simulink model "Final_PV1"  (R2015a)
settings: Solver=ode45  StartTime=0.0  StopTime=.08  MinStep=.00001  RelTol=1e-6
undefined symbols (not defined in the file): sigbuilder_block
libraries: powerlib x8, simulink x2
settings Model: Creator=TCM  LastModifiedBy=pc
settings SolverCC: ZeroCrossControl=EnableAll
settings DebuggingCC: UnderspecifiedInitializationDetection=Classic  MergeDetectMultiDrivingBlocksExec=none  SolverPrmCheckMsg=warning  StateNameClashWarn=warning

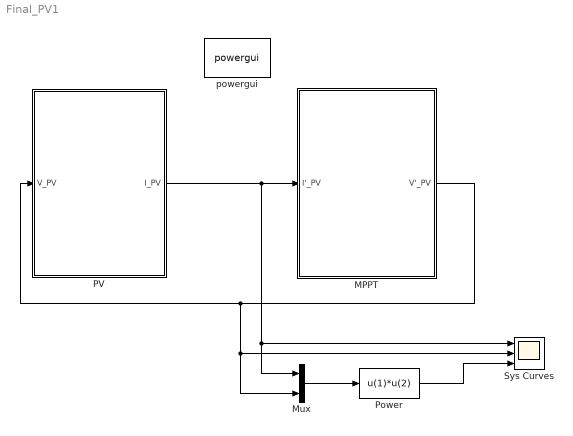
== system Final_PV1 ==
  MPPT : Subsystem
  Mux : Mux  Inputs=2
  PV : Subsystem
  "Power " : Fcn  Expr=u(1)*u(2)
  Sys Curves : Scope  NumInputPorts=3
      settings: YMin=0~0~6.15  YMax=400~80~6.4  SaveName=ScopeData2
  powergui : powerlib/powergui  Priority=1  SimulationMode=Discrete  SolverType=Tustin  SampleTime=50e-6  frequency=60  SPID=on  DisableSnubberDevices=off  DisableRonSwitches=off  DisableVfSwitches=off  SwTol=0  DisplayEquations=off  Interpol=off  methode=off  Ts=100  FunctionMessages=off  echomessages=off  HookPort=off  EnableUseOfTLC=off  x0status=blocks  frequencyindice=0  Pbase=100e6  ErrMax=1e-4  Iterations=50  UnitsV=kV  UnitsW=MW  buscounter=0  RestoreLinks=warning  ResistiveCurrentMeasurement=off  Frange=[0:2:500]  Ylog=off  Xlog=on  ShowGrid=off  save=off  variable=ZData  structure=0  ZoomFFT=off  StartTime=0.0  cycles=1  DisplayStyle=1  fundamental=60  FreqAxis=off  MaxFrequency=1000  frequencyindicesteady=1  RmsSteady=1  display=off
  wires:
  PV/1(I_PV) -> MPPT/1(I'_PV), Sys Curves/1, Mux/1
  Mux/1 -> "Power "/1
  "Power "/1 -> Sys Curves/3
  MPPT/1("V'_PV ") -> Mux/2, Sys Curves/2, PV/1(V_PV)

== system Final_PV1/MPPT ==
  I'_PV : Inport
  "MPPT " : Subsystem
  "V'_PV " : Outport
  wires:
  "MPPT "/1(V_mpp) -> "V'_PV "/1, "MPPT "/2(V_PV)
  I'_PV/1 -> "MPPT "/1(I_PV)

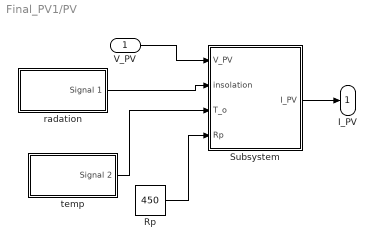
== system Final_PV1/PV ==
  V_PV : Inport
  Rp : Constant  Value=450
  Subsystem : Subsystem
  radation : Subsystem  Tag=STV Subsys  LoadFcn=sigbuilder_block('load');  StartFcn=sigbuilder_block('start');  StopFcn=sigbuilder_block('stop');  ClipboardFcn=sigbuilder_block('clipboard');  mask(Sigbuilder block){}
      mask help: Simulink:masks:SigbuilderBlock_MD
      mask init:
      | if ~strcmp(get_param(bdroot(gcbh),'SimulationStatus'),'stopped') tuvar = sigbuilder_block('maskInit'); end
      settings: CopyFcn=sigbuilder_block('copy');  DeleteFcn=sigbuilder_block('delete');  ModelCloseFcn=sigbuilder_block('modelClose');  PreSaveFcn=sigbuilder_block('preSave');  PauseFcn=sigbuilder_block('pause');  ContinueFcn=sigbuilder_block('continue');  NameChangeFcn=sigbuilder_block('namechange');  OpenFcn=sigbuilder_block('open',[267 58.5 550.5 394.5 ]);  CloseFcn=sigbuilder_block('close');
      mask Display: plot(0, 0, 100, 100,[2, 2, 32, 32, 2], [68, 8, 8, 68, 68],[32, 2], [38, 38], [32, 19, 2],[53, 60, 44], [32, 17, 17, 2],[16, 16, 31, 31]);txt = getActiveGroup(gcbh);text(2, 100, txt,'verticalAlignment', 'top');
  temp : Subsystem  Tag=STV Subsys  LoadFcn=sigbuilder_block('load');  StartFcn=sigbuilder_block('start');  StopFcn=sigbuilder_block('stop');  ClipboardFcn=sigbuilder_block('clipboard');  mask(Sigbuilder block){}
      mask help: Simulink:masks:SigbuilderBlock_MD
      mask init:
      | if ~strcmp(get_param(bdroot(gcbh),'SimulationStatus'),'stopped') tuvar = sigbuilder_block('maskInit'); end
      settings: CopyFcn=sigbuilder_block('copy');  DeleteFcn=sigbuilder_block('delete');  ModelCloseFcn=sigbuilder_block('modelClose');  PreSaveFcn=sigbuilder_block('preSave');  PauseFcn=sigbuilder_block('pause');  ContinueFcn=sigbuilder_block('continue');  NameChangeFcn=sigbuilder_block('namechange');  OpenFcn=sigbuilder_block('open',[437.25 118.5 550.5 394.5 ]);  CloseFcn=sigbuilder_block('close');
      mask Display: plot(0, 0, 100, 100,[2, 2, 32, 32, 2], [68, 8, 8, 68, 68],[32, 2], [38, 38], [32, 19, 2],[53, 60, 44], [32, 17, 17, 2],[16, 16, 31, 31]);txt = getActiveGroup(gcbh);text(2, 100, txt,'verticalAlignment', 'top');
  I_PV : Outport
  wires:
  Subsystem/1(I_PV) -> I_PV/1
  temp/1(Signal 2) -> Subsystem/3(T_o)
  radation/1(Signal 1) -> Subsystem/2(insolation)
  Rp/1 -> Subsystem/4(Rp)
  V_PV/1 -> Subsystem/1(V_PV)

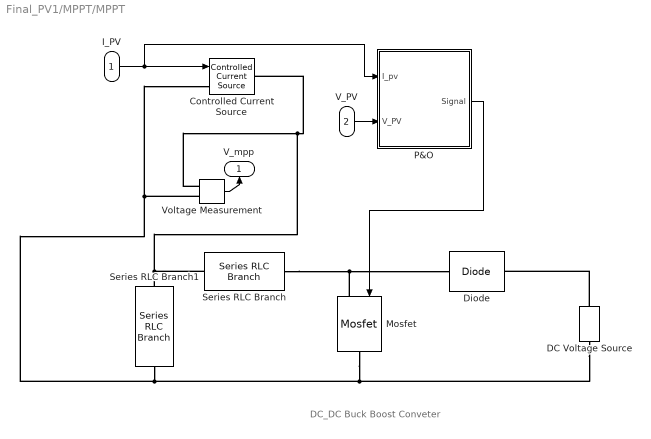
== system Final_PV1/MPPT/MPPT  ==
  note: DC_DC Buck Boost Conveter
  I_PV : Inport
  V_PV : Inport  Port=2
  Controlled Current Source : powerlib/Electrical Sources/Controlled Current Source  Initialize=on  Source_Type=AC  Amplitude=0  Phase=0  Frequency=0  Measurements=None
  DC Voltage Source : powerlib/Electrical Sources/DC Voltage Source  Amplitude=55  Measurements=None
  Diode : powerlib/Power Electronics/Diode  Ron=0.001  Lon=0  Vf=0.8  IC=0  UseSnubber=off  Rs=500  Cs=250e-9  Measurements=off
  Mosfet : powerlib/Power Electronics/Mosfet  Ron=0.1  Lon=0  Rd=0.01  Vfd=0  IC=0  Rs=1e5  Cs=inf  Measurements=off
  "P&O " : Subsystem
  Series RLC Branch : powerlib/Elements/Series RLC Branch  LConnTagsString=__new0  RConnTagsString=__new0  BranchType=RL  Resistance=.45  Inductance=1e-3  SetiL0=off  InitialCurrent=0  Capacitance=1e-6  Setx0=off  InitialVoltage=0  Measurements=None
  Series RLC Branch1 : powerlib/Elements/Series RLC Branch  LConnTagsString=__new0  RConnTagsString=__new0  BranchType=C  Resistance=1  Inductance=1e-3  SetiL0=off  InitialCurrent=0  Capacitance=2e-3  Setx0=off  InitialVoltage=0  Measurements=None
  Voltage Measurement : powerlib/Measurements/Voltage Measurement  PhasorSimulation=off  OutputType=Complex  PSBequivalent=0
  V_mpp : Outport
  wires:
  Voltage Measurement/1 -> V_mpp/1
  I_PV/1 -> "P&O "/1(I_pv), Controlled Current Source/1
  V_PV/1 -> "P&O "/2(V_PV)
  "P&O "/1(Signal) -> Mosfet/1
  connections:
  Series RLC Branch/RConn1 -- Mosfet/LConn1 -- Diode/LConn1
  Voltage Measurement/LConn1 -- Series RLC Branch/LConn1 -- Series RLC Branch1/LConn1 -- Controlled Current Source/RConn1
  Voltage Measurement/LConn2 -- DC Voltage Source/LConn1 -- Mosfet/RConn1 -- Series RLC Branch1/RConn1 -- Controlled Current Source/LConn1
  DC Voltage Source/RConn1 -- Diode/RConn1

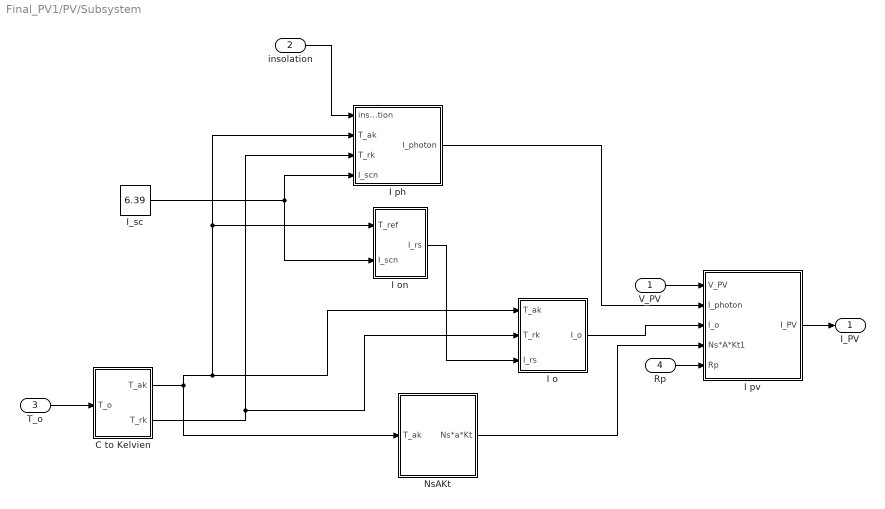
== system Final_PV1/PV/Subsystem ==
  V_PV : Inport
  insolation : Inport  Port=2
  T_o : Inport  Port=3
  Rp : Inport  Port=4
  C to Kelvien : Subsystem
  I o : Subsystem
  I on : Subsystem
  I ph : Subsystem
  I pv : Subsystem
  I_sc : Constant  Value=6.39
  NsAKt : Subsystem
  I_PV : Outport
  wires:
  T_o/1 -> C to Kelvien/1(T_o)
  insolation/1 -> I ph/1(insolation)
  C to Kelvien/2(T_rk) -> I ph/3(T_rk), I o/2(T_rk)
  I_sc/1 -> I ph/4(I_scn), I on/2(I_scn)
  NsAKt/1(Ns*a*Kt) -> I pv/4(Ns*A*Kt1)
  I on/1(I_rs) -> I o/3(I_rs)
  C to Kelvien/1(T_ak) -> I ph/2(T_ak), I on/1(T_ref), I o/1(T_ak), NsAKt/1(T_ak)
  I ph/1(I_photon) -> I pv/2(I_photon)
  I pv/1(I_PV) -> I_PV/1
  I o/1(I_o) -> I pv/3(I_o)
  V_PV/1 -> I pv/1(V_PV)
  Rp/1 -> I pv/5(Rp)

== system Final_PV1/PV/radation ==
  Demux : Demux  Tag=STV Demux  Outputs=1
  FromWs : FromWorkspace  Tag=STV FromWs  VariableName=tuvar  SampleTime=0
      SigBuilderData=|
      | common.afterFinalStr = 'Extrapolate'
      | common.sampleTime = 0
      | dataSet.timeRange = [0 10]
      | dataSet.name = 'Group 1'
      | sbobj.Groups.Name = 'Group 1'
      | sbobj.Groups.Signals.Name = 'Signal 1'
      | sbobj.Groups.Signals.XData = [0 0.05 0.05 10]
      | sbobj.Groups.Signals.YData = [1 1 0.5 0.5]
  Signal 1 : Outport  Tag=STV Outport
  wires:
  FromWs/1 -> Demux/1
  Demux/1 -> Signal 1/1

== system Final_PV1/PV/temp ==
  Demux : Demux  Tag=STV Demux  Outputs=1
  FromWs : FromWorkspace  Tag=STV FromWs  VariableName=tuvar  SampleTime=0
      SigBuilderData=|
      | common.afterFinalStr = 'Extrapolate'
      | common.sampleTime = 0
      | dataSet.timeRange = [0 10]
      | dataSet.name = 'Group 1'
      | sbobj.Groups.Name = 'Group 1'
      | sbobj.Groups.Signals.Name = 'Signal 2'
      | sbobj.Groups.Signals.XData = [0 1 2 10]
      | sbobj.Groups.Signals.YData = [25 25 25 25]
  Signal 2 : Outport  Tag=STV Outport
  wires:
  FromWs/1 -> Demux/1
  Demux/1 -> Signal 2/1

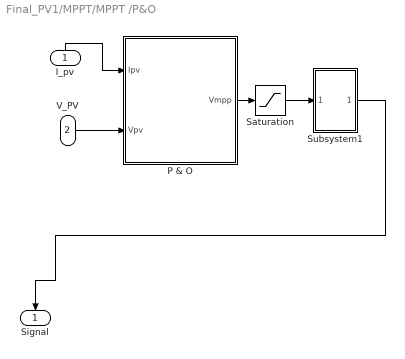
== system Final_PV1/MPPT/MPPT /P&O  ==
  I_pv : Inport
  V_PV : Inport  Port=2
  P & O : Subsystem
  Saturation : Saturate  UpperLimit=1
  Subsystem1 : Subsystem
  Signal : Outport
  wires:
  P & O/1(Vmpp) -> Saturation/1
  V_PV/1 -> P & O/2(Vpv)
  Saturation/1 -> Subsystem1/1(In1)
  Subsystem1/1(Out1) -> Signal/1
  I_pv/1 -> P & O/1(Ipv)

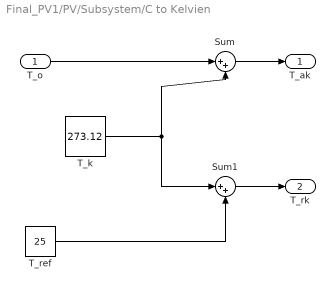
== system Final_PV1/PV/Subsystem/C to Kelvien ==
  T_o : Inport
  Sum : Sum  Inputs=|++
  Sum1 : Sum  Inputs=|++
  T_k : Constant  Value=273.12
  T_ref : Constant  Value=25
  T_ak : Outport
  T_rk : Outport  Port=2
  wires:
  T_k/1 -> Sum1/1, Sum/2
  T_o/1 -> Sum/1
  T_ref/1 -> Sum1/2
  Sum/1 -> T_ak/1
  Sum1/1 -> T_rk/1

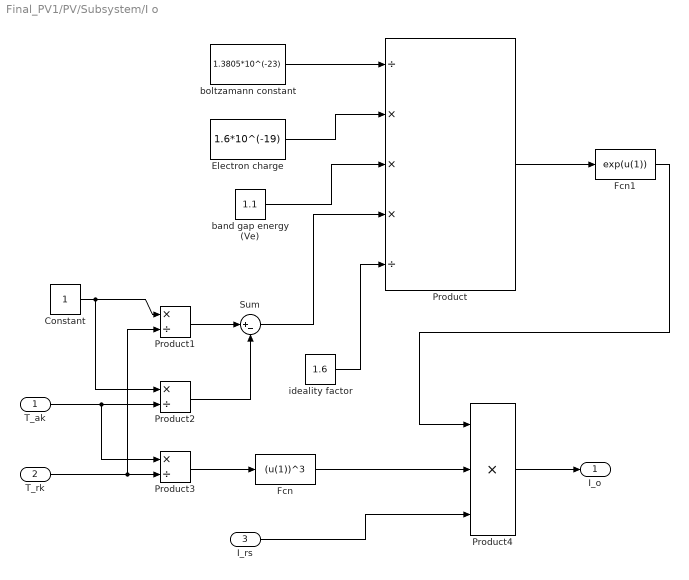
== system Final_PV1/PV/Subsystem/I o ==
  T_ak : Inport
  T_rk : Inport  Port=2
  I_rs : Inport  Port=3
  Constant : Constant
  Electron charge : Constant  Value=1.6*10^(-19)
  Fcn : Fcn  Expr=(u(1))^3
  Fcn1 : Fcn  Expr=exp(u(1))
  Product : Product  Inputs=/***/
  Product1 : Product  Inputs=*/
  Product2 : Product  Inputs=*/
  Product3 : Product  Inputs=*/
  Product4 : Product  Inputs=3
  Sum : Sum  Inputs=|+-
  band gap energy (Ve) : Constant  Value=1.1
  boltzamann constant : Constant  Value=1.3805*10^(-23)
  ideality factor : Constant  Value=1.6
  I_o : Outport
  wires:
  Electron charge/1 -> Product/2
  boltzamann constant/1 -> Product/1
  Product2/1 -> Sum/2
  I_rs/1 -> Product4/3
  band gap energy (Ve)/1 -> Product/3
  Sum/1 -> Product/4
  Product3/1 -> Fcn/1
  Product1/1 -> Sum/1
  Constant/1 -> Product2/1, Product1/1
  ideality factor/1 -> Product/5
  T_ak/1 -> Product3/1, Product2/2
  Fcn/1 -> Product4/2
  Product/1 -> Fcn1/1
  Fcn1/1 -> Product4/1
  T_rk/1 -> Product1/2, Product3/2
  Product4/1 -> I_o/1

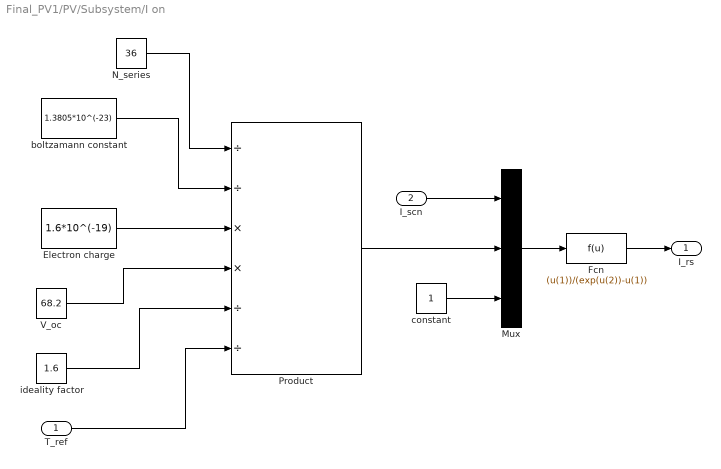
== system Final_PV1/PV/Subsystem/I on ==
  T_ref : Inport
  I_scn : Inport  Port=2
  Electron charge : Constant  Value=1.6*10^(-19)
  Fcn : Fcn  Expr=(u(1))/(exp(u(2))-u(1))
  Mux : Mux  Inputs=3
  N_series : Constant  Value=36
  Product : Product  Inputs=//**//
  V_oc : Constant  Value=68.2
  boltzamann constant : Constant  Value=1.3805*10^(-23)
  constant : Constant
  ideality factor : Constant  Value=1.6
  I_rs : Outport
  wires:
  N_series/1 -> Product/1
  boltzamann constant/1 -> Product/2
  Electron charge/1 -> Product/3
  ideality factor/1 -> Product/5
  V_oc/1 -> Product/4
  T_ref/1 -> Product/6
  Product/1 -> Mux/2
  I_scn/1 -> Mux/1
  constant/1 -> Mux/3
  Mux/1 -> Fcn/1
  Fcn/1 -> I_rs/1

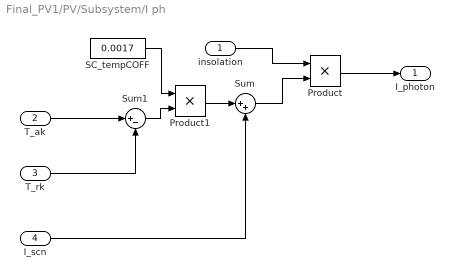
== system Final_PV1/PV/Subsystem/I ph ==
  insolation : Inport
  T_ak : Inport  Port=2
  T_rk : Inport  Port=3
  I_scn : Inport  Port=4
  Product : Product
  Product1 : Product
  SC_tempCOFF : Constant  Value=0.0017
  Sum : Sum  Inputs=|++
  Sum1 : Sum  Inputs=|+-
  I_photon : Outport
  wires:
  Product/1 -> I_photon/1
  insolation/1 -> Product/1
  T_ak/1 -> Sum1/1
  T_rk/1 -> Sum1/2
  Sum/1 -> Product/2
  I_scn/1 -> Sum/2
  Product1/1 -> Sum/1
  SC_tempCOFF/1 -> Product1/1
  Sum1/1 -> Product1/2

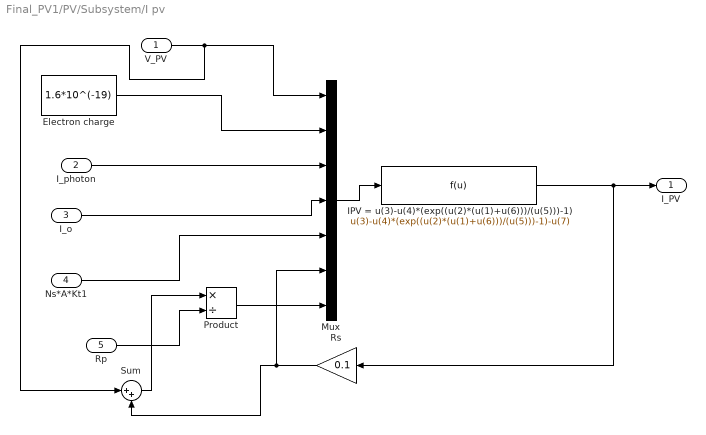
== system Final_PV1/PV/Subsystem/I pv ==
  V_PV : Inport
  I_photon : Inport  Port=2
  I_o : Inport  Port=3
  Ns*A*Kt1 : Inport  Port=4
  Rp : Inport  Port=5
  Electron charge : Constant  Value=1.6*10^(-19)
  IPV = u(3)-u(4)*(exp((u(2)*(u(1)+u(6)))/(u(5)))-1) : Fcn  Expr=u(3)-u(4)*(exp((u(2)*(u(1)+u(6)))/(u(5)))-1)-u(7)
  Mux : Mux  Inputs=7
  Product : Product  Inputs=*/
  Rs : Gain  Gain=0.1
  Sum : Sum  Inputs=|++
  I_PV : Outport
  wires:
  IPV = u(3)-u(4)*(exp((u(2)*(u(1)+u(6)))/(u(5)))-1)/1 -> I_PV/1, Rs/1
  Ns*A*Kt1/1 -> Mux/5
  Mux/1 -> IPV = u(3)-u(4)*(exp((u(2)*(u(1)+u(6)))/(u(5)))-1)/1
  I_o/1 -> Mux/4
  Rs/1 -> Sum/2, Mux/6
  Electron charge/1 -> Mux/2
  I_photon/1 -> Mux/3
  V_PV/1 -> Sum/1, Mux/1
  Sum/1 -> Product/1
  Rp/1 -> Product/2
  Product/1 -> Mux/7

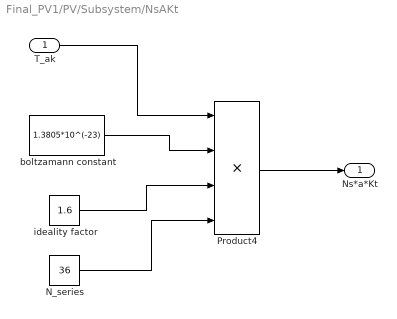
== system Final_PV1/PV/Subsystem/NsAKt ==
  T_ak : Inport
  N_series : Constant  Value=36
  Product4 : Product  Inputs=4
  boltzamann constant : Constant  Value=1.3805*10^(-23)
  ideality factor : Constant  Value=1.6
  Ns*a*Kt : Outport
  wires:
  Product4/1 -> Ns*a*Kt/1
  boltzamann constant/1 -> Product4/2
  ideality factor/1 -> Product4/3
  T_ak/1 -> Product4/1
  N_series/1 -> Product4/4

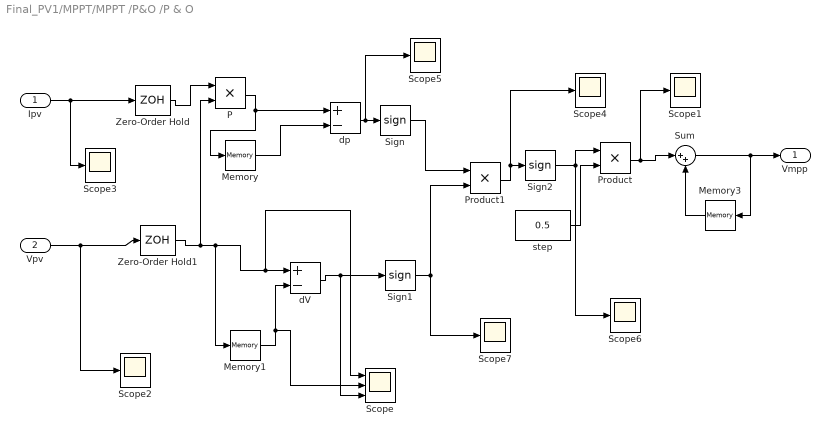
== system Final_PV1/MPPT/MPPT /P&O /P & O ==
  Ipv : Inport
  Vpv : Inport  Port=2
  Memory : Memory  InheritSampleTime=on
  Memory1 : Memory  InheritSampleTime=on
  Memory3 : Memory  InheritSampleTime=on
  P : Product  RndMeth=Zero
  Product : Product  RndMeth=Zero
  Product1 : Product  RndMeth=Zero
  Scope : Scope  NumInputPorts=3
      settings: YMin=29.1717~29.1717~1e-006  YMax=32.2424~32.2424~1.7e-005
  Scope{1..7} (7 alike) : Scope
      Scope1 settings: YMin=-0.0005  YMax=0.0005  SaveName=ScopeData34
      Scope2 settings: YMin=-11  YMax=10  SaveName=ScopeData35
      Scope3 settings: YMin=-11  YMax=10  SaveName=ScopeData36
      Scope4 settings: YMin=-11  YMax=10  SaveName=ScopeData37
      Scope5 settings: YMin=-11  YMax=10
      Scope6 settings: YMin=-11  YMax=10  SaveName=ScopeData38
      Scope7 settings: YMin=-11  YMax=10  SaveName=ScopeData39
  Sign : Signum
  Sign1 : Signum
  Sign2 : Signum
  Sum : Sum  Inputs=|++
  Zero-Order Hold : ZeroOrderHold  SampleTime=0.002
  Zero-Order Hold1 : ZeroOrderHold  SampleTime=0.002
  dV : Sum  Inputs=+-
  dp : Sum  Inputs=+-
  step : Constant  Value=0.5
  Vmpp : Outport
  wires:
  Memory1/1 -> dV/2, Scope/2
  Memory/1 -> dp/2
  Vpv/1 -> Zero-Order Hold1/1, Scope2/1
  dV/1 -> Sign1/1, Scope/3
  step/1 -> Product/2
  Product/1 -> Sum/1, Scope1/1
  Sign/1 -> Product1/1
  Sign1/1 -> Product1/2, Scope7/1
  Product1/1 -> Sign2/1, Scope4/1
  Ipv/1 -> Zero-Order Hold/1, Scope3/1
  Zero-Order Hold1/1 -> P/2, dV/1, Scope/1, Memory1/1
  Zero-Order Hold/1 -> P/1
  P/1 -> Memory/1, dp/1
  dp/1 -> Sign/1, Scope5/1
  Sign2/1 -> Product/1, Scope6/1
  Sum/1 -> Memory3/1, Vmpp/1
  Memory3/1 -> Sum/2

== system Final_PV1/MPPT/MPPT /P&O /Subsystem1 ==
  In1 : Inport
  Compare To Zero : simulink/Logic and Bit Operations/Compare To Zero  relop=<=  OutDataTypeStr=boolean
  Repeating Sequence : simulink/Sources/Repeating Sequence  rep_seq_t=[0 0.1e-3]  rep_seq_y=[0 1]
  Subtract : Sum  Inputs=+-
  Out1 : Outport
  wires:
  Compare To Zero/1 -> Out1/1
  Subtract/1 -> Compare To Zero/1
  Repeating Sequence/1 -> Subtract/2
  In1/1 -> Subtract/1
